simulink library "asbCubeSatDynamicsLib"  (R2025b)
settings: Solver=VariableStepAuto  StartTime=0.0  StopTime=10.0  RelTol=1e-3
libraries: aerolibutil x3, simulink_extras x2, sharedtransform x2, aerolibattitudesys x1, aerolibtransform2 x1
settings Model: Creator=The MathWorks, Inc.  LastModifiedBy=The MathWorks, Inc.
settings SolverCC: AlgebraicLoopSolver=TrustRegion  MaxZcPerStep=1.0
settings DataIOCC: ReturnWorkspaceOutputs=off
settings DebuggingCC: UnconnectedInputMsg=warning  UnconnectedOutputMsg=warning  UnconnectedLineMsg=warning  ArithmeticOperatorsInVariantConditions=warning
settings ModelReferenceCC: EnableRefExpFcnMdlSchedulingChecks=on
settings RTWCC: GPUComputeCapability=3.5  DLArmComputeVersion=19.05

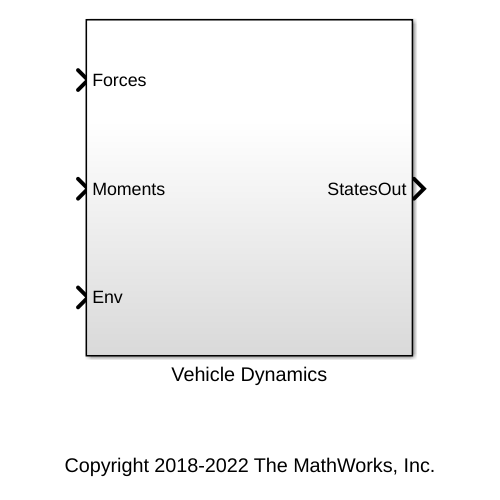
[thumbnail: Simulink's stored preview of the top-level diagram]
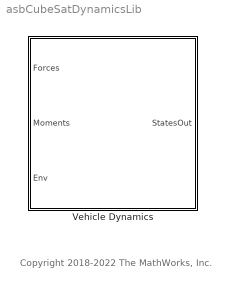
== system asbCubeSatDynamicsLib ==
  note: Copyright 2018-2022 The MathWorks, Inc.
  Vehicle Dynamics : Subsystem

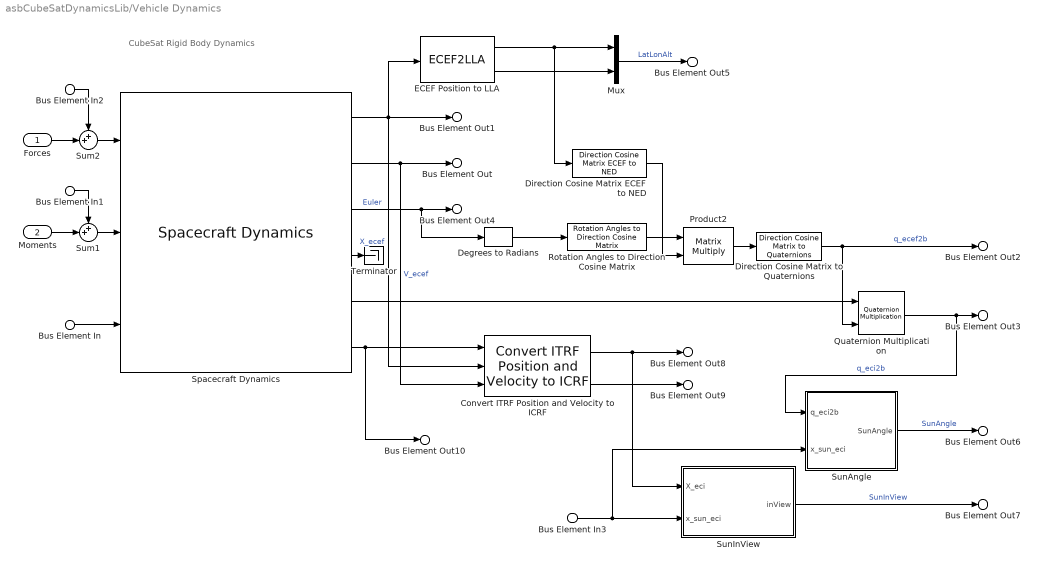
== system asbCubeSatDynamicsLib/Vehicle Dynamics ==
  note: CubeSat Rigid Body Dynamics
  Forces : Inport  RequirementInfo={} %GIDa_ddd740cf_b998_4d50_bb9f_dead4dfb86ef
  Moments : Inport  RequirementInfo={} %GIDa_0e265085_ad05_44f5_915a_efdf50105eef  Port=2
  Bus Element In : Inport  Port=3  PortName=Env  Element=envAccel_ecef
  Bus Element In1 : Inport  Port=3  PortName=Env  Element=envTorques_body
  Bus Element In2 : Inport  Port=3  PortName=Env  Element=envForces_body
  Bus Element In3 : Inport  Port=3  PortName=Env  Element=x_sun_eci
  Convert ITRF Position and Velocity to ICRF : aerolibattitudesys/Convert ITRF Position and Velocity to ICRF
  Degrees to Radians : simulink_extras/Transformations/Degrees to Radians
  Direction Cosine Matrix ECEF to NED : aerolibtransform2/Direction Cosine Matrix ECEF to NED
  Direction Cosine Matrix to Quaternions : sharedtransform/Direction Cosine Matrix  to Quaternions  RequirementInfo={} %GIDa_3db19a8f_c925_4b51_9699_85867176506c  aMode=aMode  action=None  tolerance=eps(2)
  ECEF Position to LLA : ECEF2LLA
  Mux : Mux  Inputs=2
  Product2 : Product  Multiplication=Matrix(*)  RndMeth=Zero
  Quaternion Multiplication : aerolibutil/Quaternion Multiplication
  Rotation Angles to Direction Cosine Matrix : sharedtransform/Rotation Angles to Direction Cosine Matrix  rotationOrder=ZYX  aMode=aMode
  Spacecraft Dynamics : SpacecraftDynamics  accelIn=on  accelFrame=Fixed-frame  outportFrame=Fixed-frame  startDate=initCond.simStartDate.JD  mass=vehicle.mass  inertia=vehicle.inertia  stateFormatNum=ICRF state vector  inertialPosition=initCond.r_eci  inertialVelocity=initCond.v_eci  attitudeFrame=NED  attitudeFormat=Euler angles  attitude=initCond.euler  attitudeRate=initCond.pqr  outputTransform=on
  Sum1 : Sum  RequirementInfo={} %GIDa_57348fbd_ab1f_48c5_b399_5b65774ef7a8  Inputs=++|
  Sum2 : Sum  RequirementInfo={} %GIDa_1dfe2da7_e995_414b_aa51_4201cbd27953  Inputs=++|
  SunAngle : Subsystem
  SunInView : Subsystem
  Terminator : Terminator
  Bus Element Out10 : Outport  VectorParamsAs1DForOutWhenUnconnected=off  PortName=StatesOut  Element=utc_JD
  Bus Element Out1 : Outport  VectorParamsAs1DForOutWhenUnconnected=off  PortName=StatesOut  Element=X_ecef
  Bus Element Out : Outport  VectorParamsAs1DForOutWhenUnconnected=off  PortName=StatesOut  Element=V_ecef
  Bus Element Out8 : Outport  VectorParamsAs1DForOutWhenUnconnected=off  PortName=StatesOut  Element=X_eci
  Bus Element Out9 : Outport  VectorParamsAs1DForOutWhenUnconnected=off  PortName=StatesOut  Element=V_eci
  Bus Element Out2 : Outport  VectorParamsAs1DForOutWhenUnconnected=off  PortName=StatesOut  Element=q_ecef2b
  Bus Element Out3 : Outport  VectorParamsAs1DForOutWhenUnconnected=off  PortName=StatesOut  Element=q_eci2b
  Bus Element Out4 : Outport  VectorParamsAs1DForOutWhenUnconnected=off  PortName=StatesOut  Element=Euler
  Bus Element Out5 : Outport  VectorParamsAs1DForOutWhenUnconnected=off  PortName=StatesOut  Element=LatLonAlt
  Bus Element Out6 : Outport  VectorParamsAs1DForOutWhenUnconnected=off  PortName=StatesOut  Element=SunAngle
  Bus Element Out7 : Outport  VectorParamsAs1DForOutWhenUnconnected=off  PortName=StatesOut  Element=SunInView
  wires:
  Quaternion Multiplication/1 -> SunAngle/1(q_eci2b), Bus Element Out3/1  "q_eci2b"
  ECEF Position to LLA/2 -> Mux/2
  Bus Element In1/1 -> Sum1/1
  Spacecraft Dynamics/1 -> Bus Element Out1/1, Convert ITRF Position and Velocity to ICRF/2, ECEF Position to LLA/1  "X_ecef"
  Direction Cosine Matrix to Quaternions/1 -> Bus Element Out2/1, Quaternion Multiplication/2  "q_ecef2b"
  Mux/1 -> Bus Element Out5/1  "LatLonAlt"
  Spacecraft Dynamics/3 -> Degrees to Radians/1, Bus Element Out4/1  "Euler"
  Bus Element In/1 -> Spacecraft Dynamics/3
  Forces/1 -> Sum2/2
  Moments/1 -> Sum1/2
  Sum1/1 -> Spacecraft Dynamics/2
  Spacecraft Dynamics/2 -> Bus Element Out/1, Convert ITRF Position and Velocity to ICRF/3  "V_ecef"
  Direction Cosine Matrix ECEF to NED/1 -> Product2/2
  Rotation Angles to Direction Cosine Matrix/1 -> Product2/1
  ECEF Position to LLA/1 -> Mux/1, Direction Cosine Matrix ECEF to NED/1
  Product2/1 -> Direction Cosine Matrix to Quaternions/1
  Spacecraft Dynamics/5 -> Quaternion Multiplication/1
  Spacecraft Dynamics/4 -> Terminator/1
  Spacecraft Dynamics/6 -> Bus Element Out10/1, Convert ITRF Position and Velocity to ICRF/1
  Degrees to Radians/1 -> Rotation Angles to Direction Cosine Matrix/1
  Sum2/1 -> Spacecraft Dynamics/1
  Bus Element In2/1 -> Sum2/1
  SunAngle/1(SunAngle) -> Bus Element Out6/1  "SunAngle"
  Bus Element In3/1 -> SunAngle/2(x_sun_eci), SunInView/2(x_sun_eci)
  SunInView/1(inView) -> Bus Element Out7/1  "SunInView"
  Convert ITRF Position and Velocity to ICRF/1 -> Bus Element Out8/1, SunInView/1(X_eci)
  Convert ITRF Position and Velocity to ICRF/2 -> Bus Element Out9/1

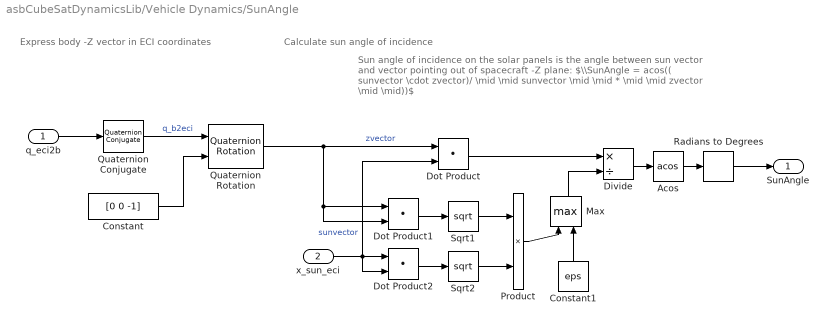
== system asbCubeSatDynamicsLib/Vehicle Dynamics/SunAngle ==
  note: Express body -Z vector in ECI coordinates
  note: Calculate sun angle of incidence
  note: Sun angle of incidence on the solar panels is the angle between sun vector and vector pointing out of spacecraft -Z plane:
      | $\\SunAngle = acos(( sunvector \cdot zvector)/ \mid \mid sunvector \mid \mid * \mid \mid zvector \mid \mid))$
  q_eci2b : Inport  SampleTime=0
  x_sun_eci : Inport  Port=2  SampleTime=0
  Acos : Trigonometry  Operator=acos
  Constant : Constant  Value=[0 0 -1]  SampleTime=0
  Constant1 : Constant  Value=eps
  Divide : Product  Inputs=*/
  Dot Product : DotProduct  OutDataTypeStr=Inherit: Inherit via internal rule
  Dot Product1 : DotProduct  OutDataTypeStr=Inherit: Inherit via internal rule
  Dot Product2 : DotProduct  OutDataTypeStr=Inherit: Inherit via internal rule
  Max : MinMax  Function=max  Inputs=2
  Product : Product
  Quaternion Conjugate : aerolibutil/Quaternion Conjugate
  Quaternion Rotation : aerolibutil/Quaternion Rotation
  Radians to Degrees : simulink_extras/Transformations/Radians to Degrees
  Sqrt1 : Sqrt
  Sqrt2 : Sqrt
  SunAngle : Outport  SampleTime=0
  wires:
  Radians to Degrees/1 -> SunAngle/1
  x_sun_eci/1 -> Dot Product/2, Dot Product2/2, Dot Product2/1  "sunvector"
  Dot Product/1 -> Divide/1
  Divide/1 -> Acos/1
  Acos/1 -> Radians to Degrees/1
  Dot Product1/1 -> Sqrt1/1
  Quaternion Rotation/1 -> Dot Product/1, Dot Product1/2, Dot Product1/1  "zvector"
  Constant/1 -> Quaternion Rotation/2
  q_eci2b/1 -> Quaternion Conjugate/1
  Quaternion Conjugate/1 -> Quaternion Rotation/1  "q_b2eci"
  Dot Product2/1 -> Sqrt2/1
  Sqrt1/1 -> Product/1
  Sqrt2/1 -> Product/2
  Product/1 -> Max/1
  Constant1/1 -> Max/2
  Max/1 -> Divide/2

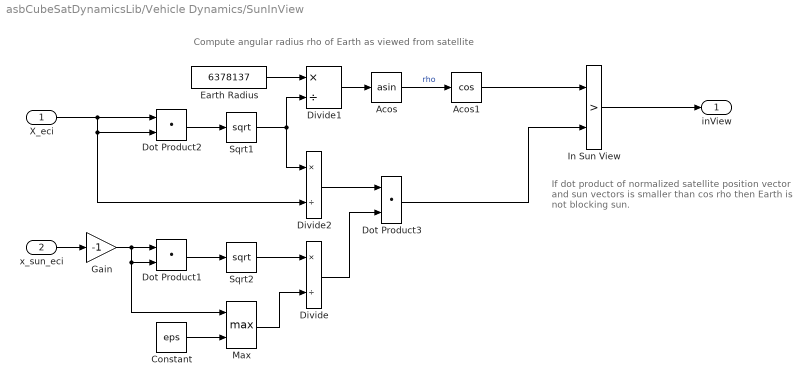
== system asbCubeSatDynamicsLib/Vehicle Dynamics/SunInView ==
  note: Compute angular radius rho of Earth as viewed from satellite
  note: If dot product of normalized satellite position vector and sun vectors is smaller than cos rho then Earth is not blocking sun.
  X_eci : Inport
  x_sun_eci : Inport  Port=2  SampleTime=0
  Acos : Trigonometry  Operator=asin
  Acos1 : Trigonometry  Operator=cos
  Constant : Constant  Value=eps
  Divide : Product  Inputs=*/
  Divide1 : Product  Inputs=*/
  Divide2 : Product  Inputs=*/
  Dot Product1 : DotProduct  OutDataTypeStr=Inherit: Inherit via internal rule
  Dot Product2 : DotProduct  OutDataTypeStr=Inherit: Inherit via internal rule
  Dot Product3 : DotProduct  OutDataTypeStr=Inherit: Inherit via internal rule
  Earth Radius : Constant  Value=6378137  VectorParams1D=off  SampleTime=0
  Gain : Gain  Gain=-1
  In Sun View : RelationalOperator  Operator=>  OutDataTypeStr=boolean  ZeroCross=off  RndMeth=Simplest  InputSameDT=off
  Max : MinMax  Function=max  Inputs=2
  Sqrt1 : Sqrt
  Sqrt2 : Sqrt
  inView : Outport  SampleTime=0
  wires:
  Gain/1 -> Max/1, Dot Product1/2, Dot Product1/1
  In Sun View/1 -> inView/1
  X_eci/1 -> Divide2/2, Dot Product2/2, Dot Product2/1
  Earth Radius/1 -> Divide1/1
  Dot Product2/1 -> Sqrt1/1
  x_sun_eci/1 -> Gain/1
  Sqrt1/1 -> Divide2/1, Divide1/2
  Divide1/1 -> Acos/1
  Acos/1 -> Acos1/1  "rho"
  Divide/1 -> Dot Product3/2
  Acos1/1 -> In Sun View/1
  Divide2/1 -> Dot Product3/1
  Dot Product3/1 -> In Sun View/2
  Sqrt2/1 -> Divide/1
  Dot Product1/1 -> Sqrt2/1
  Constant/1 -> Max/2
  Max/1 -> Divide/2
